simulink model "UserDefinedModel"  (R2023b)
settings: Solver=ode45  StartTime=0.0  StopTime=20  MaxStep=0.001  RelTol=1e-3
libraries: spsSeriesRLCBranchLib x131, spsGroundLib x55, spsCurrentMeasurementLib x48, spsVoltageMeasurementLib x17, spsDiodeLib x4, spsControlledVoltageSourceLib x2, spspowerguiLib x1
(part 1 of 2)
settings Model: Creator=DJJ  LastModifiedBy=HP
settings SolverCC: AlgebraicLoopSolver=TrustRegion
settings DataIOCC: ReturnWorkspaceOutputs=off
settings DebuggingCC: UnconnectedInputMsg=warning  UnconnectedOutputMsg=warning  UnconnectedLineMsg=warning  ArithmeticOperatorsInVariantConditions=warning
settings ModelReferenceCC: EnableRefExpFcnMdlSchedulingChecks=on
settings SFSimCC: CustomCodeUndefinedFunction=UseInterfaceOnly

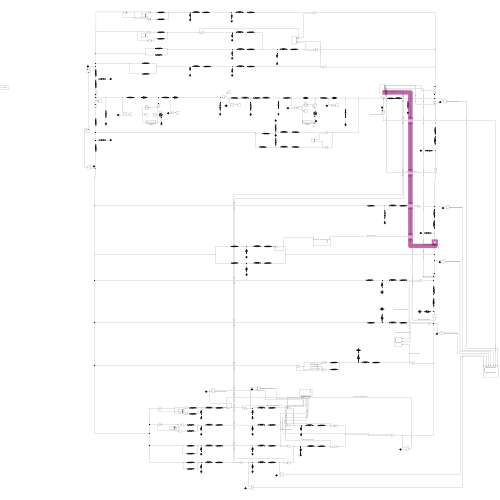
[thumbnail: Simulink's stored preview of the top-level diagram]
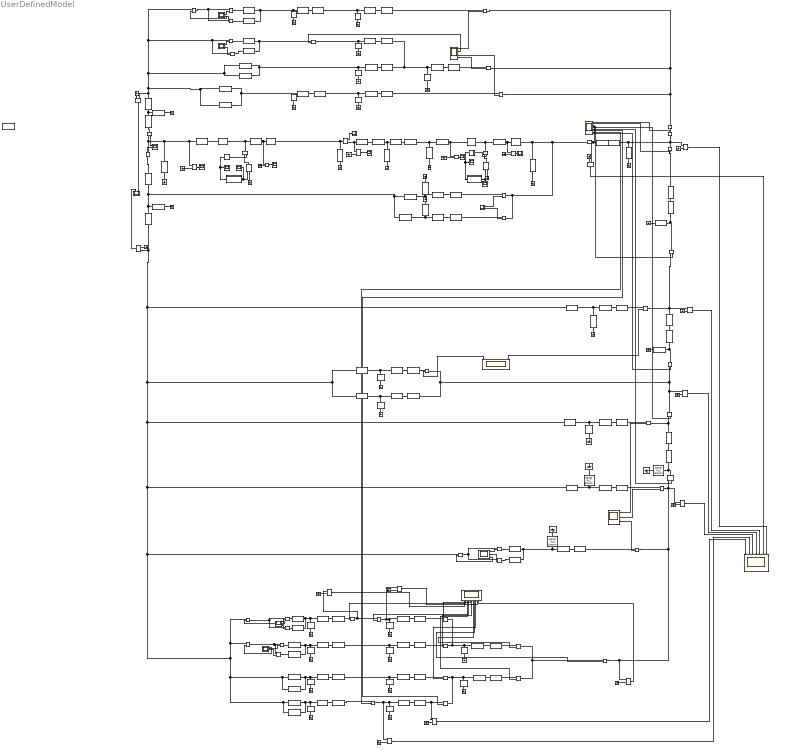
== system UserDefinedModel ==
  Controlled Voltage Source : spsControlledVoltageSourceLib/Controlled Voltage Source  Initialize=off  Source_Type=DC  Amplitude=0  Phase=0  Frequency=0  Measurements=Voltage
  Controlled Voltage Source1 : spsControlledVoltageSourceLib/Controlled Voltage Source  Initialize=off  Source_Type=DC  Amplitude=0  Phase=0  Frequency=0  Measurements=None
  Current Measurement{1,5..19,23..26,31..40,46..49,51..52,58..64,67..68} (45 alike) : spsCurrentMeasurementLib/Current Measurement  PhasorSimulation=off  OutputType=Complex  PSBequivalent=0
  Current Measurement2 : spsCurrentMeasurementLib/Current Measurement  PhasorSimulation=off  OutputType=Magnitude  PSBequivalent=0
  Current Measurement3 : spsCurrentMeasurementLib/Current Measurement  PhasorSimulation=off  OutputType=Magnitude  PSBequivalent=0
  Current Measurement4 : spsCurrentMeasurementLib/Current Measurement  PhasorSimulation=off  OutputType=Magnitude  PSBequivalent=0
  Diode1 : spsDiodeLib/Diode  Ron=0  Lon=0  Vf=0  IC=0  UseSnubber=0  Rs=inf  Cs=250e-9  Measurements=off
  Diode3 : spsDiodeLib/Diode  Ron=0.015  Lon=0  Vf=0  IC=0  UseSnubber=0  Rs=inf  Cs=250e-9  Measurements=off
  Diode5 : spsDiodeLib/Diode  Ron=0  Lon=0  Vf=0  IC=0  UseSnubber=0  Rs=inf  Cs=250e-9  Measurements=off
  Diode7 : spsDiodeLib/Diode  Ron=0.003751  Lon=0  Vf=0  IC=0  UseSnubber=0  Rs=inf  Cs=250e-9  Measurements=off
  Ground{1..30,34,36..40,42..43,47..51,54..55,58..67} (55 alike) : spsGroundLib/Ground  LConnTagsString=a
  Scope1 : Scope  NumInputPorts=5
  Scope{3,5..13} (10 alike) : Scope
  Scope14 : Scope  NumInputPorts=8
  Scope15 : Scope  NumInputPorts=2
  Scope16 : Scope  NumInputPorts=3
  Scope18 : Scope  NumInputPorts=11
  Scope2 : Scope  NumInputPorts=9
  Scope20 : Scope  NumInputPorts=3
  Scope21 : Scope  NumInputPorts=2
  Scope22 : Scope  NumInputPorts=5
  Scope23 : Scope  NumInputPorts=6
  Scope26 : Scope  NumInputPorts=7
  Scope27 : Scope  NumInputPorts=7
  Scope28 : Scope  NumInputPorts=3
  Scope4 : Scope  NumInputPorts=7
  Series RLC Branch1 : spsSeriesRLCBranchLib/Series RLC Branch  LConnTagsString=__new0  RConnTagsString=__new0  BranchType=R  Resistance=0.05  Inductance=1e-3  SetiL0=off  InitialCurrent=0  Capacitance=1e-6  Setx0=off  InitialVoltage=0  Measurements=None
  Series RLC Branch10 : spsSeriesRLCBranchLib/Series RLC Branch  LConnTagsString=__new0  RConnTagsString=__new0  BranchType=R  Resistance=0.025  Inductance=1e-3  SetiL0=off  InitialCurrent=0  Capacitance=1e-6  Setx0=off  InitialVoltage=0  Measurements=None
  Series RLC Branch11 : spsSeriesRLCBranchLib/Series RLC Branch  LConnTagsString=__new0  RConnTagsString=__new0  BranchType=L  Resistance=1  Inductance=0.001  SetiL0=off  InitialCurrent=0  Capacitance=1e-6  Setx0=off  InitialVoltage=0  Measurements=None
  Series RLC Branch110 : spsSeriesRLCBranchLib/Series RLC Branch  LConnTagsString=__new0  RConnTagsString=__new0  BranchType=R  Resistance=16.45  Inductance=1e-3  SetiL0=off  InitialCurrent=0  Capacitance=1e-6  Setx0=off  InitialVoltage=0  Measurements=None
  Series RLC Branch111 : spsSeriesRLCBranchLib/Series RLC Branch  LConnTagsString=__new0  RConnTagsString=__new0  BranchType=R  Resistance=2.5  Inductance=1e-3  SetiL0=off  InitialCurrent=0  Capacitance=1e-6  Setx0=off  InitialVoltage=0  Measurements=None
  Series RLC Branch{51,112,116,121} (4 alike) : spsSeriesRLCBranchLib/Series RLC Branch  LConnTagsString=__new0  RConnTagsString=__new0  BranchType=L  Resistance=1  Inductance=0.12  SetiL0=off  InitialCurrent=0  Capacitance=1e-6  Setx0=off  InitialVoltage=0  Measurements=None
  Series RLC Branch113 : spsSeriesRLCBranchLib/Series RLC Branch  LConnTagsString=__new0  RConnTagsString=__new0  BranchType=C  Resistance=1  Inductance=1e-3  SetiL0=off  InitialCurrent=0  Capacitance=0.05  Setx0=off  InitialVoltage=0  Measurements=None
  Series RLC Branch114 : spsSeriesRLCBranchLib/Series RLC Branch  LConnTagsString=__new0  RConnTagsString=__new0  BranchType=R  Resistance=16.45  Inductance=1e-3  SetiL0=off  InitialCurrent=0  Capacitance=1e-6  Setx0=off  InitialVoltage=0  Measurements=None
  Series RLC Branch115 : spsSeriesRLCBranchLib/Series RLC Branch  LConnTagsString=__new0  RConnTagsString=__new0  BranchType=R  Resistance=2.5  Inductance=1e-3  SetiL0=off  InitialCurrent=0  Capacitance=1e-6  Setx0=off  InitialVoltage=0  Measurements=None
  Series RLC Branch117 : spsSeriesRLCBranchLib/Series RLC Branch  LConnTagsString=__new0  RConnTagsString=__new0  BranchType=C  Resistance=1  Inductance=1e-3  SetiL0=off  InitialCurrent=0  Capacitance=0.05  Setx0=off  InitialVoltage=0  Measurements=None
  Series RLC Branch118 : spsSeriesRLCBranchLib/Series RLC Branch  LConnTagsString=__new0  RConnTagsString=__new0  BranchType=R  Resistance=0.07  Inductance=1e-3  SetiL0=off  InitialCurrent=0  Capacitance=1e-6  Setx0=off  InitialVoltage=0  Measurements=None
  Series RLC Branch119 : spsSeriesRLCBranchLib/Series RLC Branch  LConnTagsString=__new0  RConnTagsString=__new0  BranchType=L  Resistance=1  Inductance=0.0028  SetiL0=off  InitialCurrent=0  Capacitance=1e-6  Setx0=off  InitialVoltage=0  Measurements=None
  Series RLC Branch12 : spsSeriesRLCBranchLib/Series RLC Branch  LConnTagsString=__new0  RConnTagsString=__new0  BranchType=C  Resistance=1  Inductance=1e-3  SetiL0=off  InitialCurrent=0  Capacitance=3  Setx0=on  InitialVoltage=13.392  Measurements=None
  Series RLC Branch120 : spsSeriesRLCBranchLib/Series RLC Branch  LConnTagsString=__new0  RConnTagsString=__new0  BranchType=R  Resistance=1.5  Inductance=1e-3  SetiL0=off  InitialCurrent=0  Capacitance=1e-6  Setx0=off  InitialVoltage=0  Measurements=None
  Series RLC Branch122 : spsSeriesRLCBranchLib/Series RLC Branch  LConnTagsString=__new0  RConnTagsString=__new0  BranchType=C  Resistance=1  Inductance=1e-3  SetiL0=off  InitialCurrent=0  Capacitance=0.05  Setx0=off  InitialVoltage=0  Measurements=None
  Series RLC Branch123 : spsSeriesRLCBranchLib/Series RLC Branch  LConnTagsString=__new0  RConnTagsString=__new0  BranchType=R  Resistance=7.05  Inductance=1e-3  SetiL0=off  InitialCurrent=0  Capacitance=1e-6  Setx0=off  InitialVoltage=0  Measurements=None
  Series RLC Branch124 : spsSeriesRLCBranchLib/Series RLC Branch  LConnTagsString=__new0  RConnTagsString=__new0  BranchType=C  Resistance=1  Inductance=1e-3  SetiL0=off  InitialCurrent=0  Capacitance=0.1  Setx0=off  InitialVoltage=0  Measurements=None
  Series RLC Branch125 : spsSeriesRLCBranchLib/Series RLC Branch  LConnTagsString=__new0  RConnTagsString=__new0  BranchType=R  Resistance=4  Inductance=1e-3  SetiL0=off  InitialCurrent=0  Capacitance=1e-6  Setx0=off  InitialVoltage=0  Measurements=None
  Series RLC Branch126 : spsSeriesRLCBranchLib/Series RLC Branch  LConnTagsString=__new0  RConnTagsString=__new0  BranchType=L  Resistance=1  Inductance=0.36  SetiL0=off  InitialCurrent=0  Capacitance=1e-6  Setx0=off  InitialVoltage=0  Measurements=None
  Series RLC Branch127 : spsSeriesRLCBranchLib/Series RLC Branch  LConnTagsString=__new0  RConnTagsString=__new0  BranchType=C  Resistance=1  Inductance=1e-3  SetiL0=off  InitialCurrent=0  Capacitance=0.01  Setx0=off  InitialVoltage=0  Measurements=None
  Series RLC Branch128 : spsSeriesRLCBranchLib/Series RLC Branch  LConnTagsString=__new0  RConnTagsString=__new0  BranchType=R  Resistance=47  Inductance=1e-3  SetiL0=off  InitialCurrent=0  Capacitance=1e-6  Setx0=off  InitialVoltage=0  Measurements=None
  Series RLC Branch129 : spsSeriesRLCBranchLib/Series RLC Branch  LConnTagsString=__new0  RConnTagsString=__new0  BranchType=R  Resistance=54.58204  Inductance=1e-3  SetiL0=off  InitialCurrent=0  Capacitance=1e-6  Setx0=off  InitialVoltage=0  Measurements=None
  Series RLC Branch{5,19,87,132} (4 alike) : spsSeriesRLCBranchLib/Series RLC Branch  LConnTagsString=__new0  RConnTagsString=__new0  BranchType=R  Resistance=0.3  Inductance=1e-3  SetiL0=off  InitialCurrent=0  Capacitance=1e-6  Setx0=off  InitialVoltage=0  Measurements=None
  Series RLC Branch133 : spsSeriesRLCBranchLib/Series RLC Branch  LConnTagsString=__new0  RConnTagsString=__new0  BranchType=L  Resistance=1  Inductance=0.04  SetiL0=off  InitialCurrent=0  Capacitance=1e-6  Setx0=off  InitialVoltage=0  Measurements=None
  Series RLC Branch135 : spsSeriesRLCBranchLib/Series RLC Branch  LConnTagsString=__new0  RConnTagsString=__new0  BranchType=R  Resistance=143.364  Inductance=1e-3  SetiL0=off  InitialCurrent=0  Capacitance=1e-6  Setx0=off  InitialVoltage=0  Measurements=None
  Series RLC Branch136 : spsSeriesRLCBranchLib/Series RLC Branch  LConnTagsString=__new0  RConnTagsString=__new0  BranchType=R  Resistance=1.5  Inductance=1e-3  SetiL0=off  InitialCurrent=0  Capacitance=1e-6  Setx0=off  InitialVoltage=0  Measurements=None
  Series RLC Branch137 : spsSeriesRLCBranchLib/Series RLC Branch  LConnTagsString=__new0  RConnTagsString=__new0  BranchType=L  Resistance=1  Inductance=0.028  SetiL0=off  InitialCurrent=0  Capacitance=1e-6  Setx0=off  InitialVoltage=0  Measurements=None
  Series RLC Branch{7,138..139,143} (4 alike) : spsSeriesRLCBranchLib/Series RLC Branch  LConnTagsString=__new0  RConnTagsString=__new0  BranchType=C  Resistance=1  Inductance=1e-3  SetiL0=off  InitialCurrent=0  Capacitance=0.009  Setx0=off  InitialVoltage=0  Measurements=None
  Series RLC Branch14 : spsSeriesRLCBranchLib/Series RLC Branch  LConnTagsString=__new0  RConnTagsString=__new0  BranchType=R  Resistance=21.889  Inductance=1e-3  SetiL0=off  InitialCurrent=0  Capacitance=1e-6  Setx0=off  InitialVoltage=0  Measurements=None
  Series RLC Branch140 : spsSeriesRLCBranchLib/Series RLC Branch  LConnTagsString=__new0  RConnTagsString=__new0  BranchType=R  Resistance=143.364  Inductance=1e-3  SetiL0=off  InitialCurrent=0  Capacitance=1e-6  Setx0=off  InitialVoltage=0  Measurements=None
  Series RLC Branch141 : spsSeriesRLCBranchLib/Series RLC Branch  LConnTagsString=__new0  RConnTagsString=__new0  BranchType=R  Resistance=1.5  Inductance=1e-3  SetiL0=off  InitialCurrent=0  Capacitance=1e-6  Setx0=off  InitialVoltage=0  Measurements=None
  Series RLC Branch142 : spsSeriesRLCBranchLib/Series RLC Branch  LConnTagsString=__new0  RConnTagsString=__new0  BranchType=L  Resistance=1  Inductance=0.028  SetiL0=off  InitialCurrent=0  Capacitance=1e-6  Setx0=off  InitialVoltage=0  Measurements=None
  Series RLC Branch15 : spsSeriesRLCBranchLib/Series RLC Branch  LConnTagsString=__new0  RConnTagsString=__new0  BranchType=C  Resistance=1  Inductance=1e-3  SetiL0=off  InitialCurrent=0  Capacitance=0.038  Setx0=off  InitialVoltage=0  Measurements=None
  Series RLC Branch150 : spsSeriesRLCBranchLib/Series RLC Branch  LConnTagsString=__new0  RConnTagsString=__new0  BranchType=R  Resistance=21.889  Inductance=1e-3  SetiL0=off  InitialCurrent=0  Capacitance=1e-6  Setx0=off  InitialVoltage=0  Measurements=None
  Series RLC Branch151 : spsSeriesRLCBranchLib/Series RLC Branch  LConnTagsString=__new0  RConnTagsString=__new0  BranchType=R  Resistance=48.3677  Inductance=1e-3  SetiL0=off  InitialCurrent=0  Capacitance=1e-6  Setx0=off  InitialVoltage=0  Measurements=None
  Series RLC Branch{152,158,160,164,167,177} (6 alike) : spsSeriesRLCBranchLib/Series RLC Branch  LConnTagsString=__new0  RConnTagsString=__new0  BranchType=R  Resistance=2  Inductance=1e-3  SetiL0=off  InitialCurrent=0  Capacitance=1e-6  Setx0=off  InitialVoltage=0  Measurements=None
  Series RLC Branch153 : spsSeriesRLCBranchLib/Series RLC Branch  LConnTagsString=__new0  RConnTagsString=__new0  BranchType=L  Resistance=1  Inductance=0.03  SetiL0=off  InitialCurrent=0  Capacitance=1e-6  Setx0=off  InitialVoltage=0  Measurements=None
  Series RLC Branch154 : spsSeriesRLCBranchLib/Series RLC Branch  LConnTagsString=__new0  RConnTagsString=__new0  BranchType=C  Resistance=1  Inductance=1e-3  SetiL0=off  InitialCurrent=0  Capacitance=0.018  Setx0=off  InitialVoltage=0  Measurements=None
  Series RLC Branch155 : spsSeriesRLCBranchLib/Series RLC Branch  LConnTagsString=__new0  RConnTagsString=__new0  BranchType=R  Resistance=126.5632  Inductance=1e-3  SetiL0=off  InitialCurrent=0  Capacitance=1e-6  Setx0=off  InitialVoltage=0  Measurements=None
  Series RLC Branch159 : spsSeriesRLCBranchLib/Series RLC Branch  LConnTagsString=__new0  RConnTagsString=__new0  BranchType=L  Resistance=1  Inductance=0.15  SetiL0=off  InitialCurrent=0  Capacitance=1e-6  Setx0=off  InitialVoltage=0  Measurements=None
  Series RLC Branch16 : spsSeriesRLCBranchLib/Series RLC Branch  LConnTagsString=__new0  RConnTagsString=__new0  BranchType=R  Resistance=0.35  Inductance=1e-3  SetiL0=off  InitialCurrent=0  Capacitance=1e-6  Setx0=off  InitialVoltage=0  Measurements=None
  Series RLC Branch161 : spsSeriesRLCBranchLib/Series RLC Branch  LConnTagsString=__new0  RConnTagsString=__new0  BranchType=L  Resistance=1  Inductance=0.25  SetiL0=off  InitialCurrent=0  Capacitance=1e-6  Setx0=off  InitialVoltage=0  Measurements=None
  Series RLC Branch162 : spsSeriesRLCBranchLib/Series RLC Branch  LConnTagsString=__new0  RConnTagsString=__new0  BranchType=C  Resistance=1  Inductance=1e-3  SetiL0=off  InitialCurrent=0  Capacitance=0.006  Setx0=off  InitialVoltage=0  Measurements=None
  Series RLC Branch{74,78,94,163,166} (5 alike) : spsSeriesRLCBranchLib/Series RLC Branch  LConnTagsString=__new0  RConnTagsString=__new0  BranchType=C  Resistance=1  Inductance=1e-3  SetiL0=off  InitialCurrent=0  Capacitance=0.005  Setx0=off  InitialVoltage=0  Measurements=None
  Series RLC Branch165 : spsSeriesRLCBranchLib/Series RLC Branch  LConnTagsString=__new0  RConnTagsString=__new0  BranchType=L  Resistance=1  Inductance=0.25  SetiL0=off  InitialCurrent=0  Capacitance=1e-6  Setx0=off  InitialVoltage=0  Measurements=None
  Series RLC Branch168 : spsSeriesRLCBranchLib/Series RLC Branch  LConnTagsString=__new0  RConnTagsString=__new0  BranchType=L  Resistance=1  Inductance=0.15  SetiL0=off  InitialCurrent=0  Capacitance=1e-6  Setx0=off  InitialVoltage=0  Measurements=None
  Series RLC Branch169 : spsSeriesRLCBranchLib/Series RLC Branch  LConnTagsString=__new0  RConnTagsString=__new0  BranchType=C  Resistance=1  Inductance=1e-3  SetiL0=off  InitialCurrent=0  Capacitance=0.006  Setx0=off  InitialVoltage=0  Measurements=None
  Series RLC Branch17 : spsSeriesRLCBranchLib/Series RLC Branch  LConnTagsString=__new0  RConnTagsString=__new0  BranchType=L  Resistance=1  Inductance=0.06  SetiL0=off  InitialCurrent=0  Capacitance=1e-6  Setx0=off  InitialVoltage=0  Measurements=None
  Series RLC Branch170 : spsSeriesRLCBranchLib/Series RLC Branch  LConnTagsString=__new0  RConnTagsString=__new0  BranchType=R  Resistance=0.05  Inductance=1e-3  SetiL0=off  InitialCurrent=0  Capacitance=1e-6  Setx0=off  InitialVoltage=0  Measurements=None
  Series RLC Branch171 : spsSeriesRLCBranchLib/Series RLC Branch  LConnTagsString=__new0  RConnTagsString=__new0  BranchType=L  Resistance=1  Inductance=0.004  SetiL0=off  InitialCurrent=0  Capacitance=1e-6  Setx0=off  InitialVoltage=0  Measurements=None
  Series RLC Branch172 : spsSeriesRLCBranchLib/Series RLC Branch  LConnTagsString=__new0  RConnTagsString=__new0  BranchType=C  Resistance=1  Inductance=1e-3  SetiL0=off  InitialCurrent=0  Capacitance=0.012  Setx0=off  InitialVoltage=0  Measurements=None
  Series RLC Branch173 : spsSeriesRLCBranchLib/Series RLC Branch  LConnTagsString=__new0  RConnTagsString=__new0  BranchType=R  Resistance=0.05  Inductance=1e-3  SetiL0=off  InitialCurrent=0  Capacitance=1e-6  Setx0=off  InitialVoltage=0  Measurements=None
  Series RLC Branch174 : spsSeriesRLCBranchLib/Series RLC Branch  LConnTagsString=__new0  RConnTagsString=__new0  BranchType=L  Resistance=1  Inductance=0.004  SetiL0=off  InitialCurrent=0  Capacitance=1e-6  Setx0=off  InitialVoltage=0  Measurements=None
  Series RLC Branch175 : spsSeriesRLCBranchLib/Series RLC Branch  LConnTagsString=__new0  RConnTagsString=__new0  BranchType=C  Resistance=1  Inductance=1e-3  SetiL0=off  InitialCurrent=0  Capacitance=0.012  Setx0=off  InitialVoltage=0  Measurements=None
  Series RLC Branch176 : spsSeriesRLCBranchLib/Series RLC Branch  LConnTagsString=__new0  RConnTagsString=__new0  BranchType=R  Resistance=67.5  Inductance=1e-3  SetiL0=off  InitialCurrent=0  Capacitance=1e-6  Setx0=off  InitialVoltage=0  Measurements=None
  Series RLC Branch178 : spsSeriesRLCBranchLib/Series RLC Branch  LConnTagsString=__new0  RConnTagsString=__new0  BranchType=C  Resistance=1  Inductance=1e-3  SetiL0=off  InitialCurrent=0  Capacitance=0.0012  Setx0=off  InitialVoltage=0  Measurements=None
  Series RLC Branch179 : spsSeriesRLCBranchLib/Series RLC Branch  LConnTagsString=__new0  RConnTagsString=__new0  BranchType=L  Resistance=1  Inductance=3.5  SetiL0=off  InitialCurrent=0  Capacitance=1e-6  Setx0=off  InitialVoltage=0  Measurements=None
  Series RLC Branch18 : spsSeriesRLCBranchLib/Series RLC Branch  LConnTagsString=__new0  RConnTagsString=__new0  BranchType=R  Resistance=35.84  Inductance=1e-3  SetiL0=off  InitialCurrent=0  Capacitance=1e-6  Setx0=off  InitialVoltage=0  Measurements=None
  Series RLC Branch180 : spsSeriesRLCBranchLib/Series RLC Branch  LConnTagsString=__new0  RConnTagsString=__new0  BranchType=R  Resistance=21.15  Inductance=1e-3  SetiL0=off  InitialCurrent=0  Capacitance=1e-6  Setx0=off  InitialVoltage=0  Measurements=None
  Series RLC Branch186 : spsSeriesRLCBranchLib/Series RLC Branch  LConnTagsString=__new0  RConnTagsString=__new0  BranchType=R  Resistance=61.55214  Inductance=1e-3  SetiL0=off  InitialCurrent=0  Capacitance=1e-6  Setx0=off  InitialVoltage=0  Measurements=None
  Series RLC Branch187 : spsSeriesRLCBranchLib/Series RLC Branch  LConnTagsString=__new0  RConnTagsString=__new0  BranchType=R  Resistance=17.6218  Inductance=1e-3  SetiL0=off  InitialCurrent=0  Capacitance=1e-6  Setx0=off  InitialVoltage=0  Measurements=None
  Series RLC Branch2 : spsSeriesRLCBranchLib/Series RLC Branch  LConnTagsString=__new0  RConnTagsString=__new0  BranchType=L  Resistance=1  Inductance=0.0015  SetiL0=on  InitialCurrent=23.836  Capacitance=1e-6  Setx0=off  InitialVoltage=0  Measurements=None
  Series RLC Branch20 : spsSeriesRLCBranchLib/Series RLC Branch  LConnTagsString=__new0  RConnTagsString=__new0  BranchType=L  Resistance=1  Inductance=0.005  SetiL0=off  InitialCurrent=0  Capacitance=1e-6  Setx0=off  InitialVoltage=0  Measurements=None
  Series RLC Branch21 : spsSeriesRLCBranchLib/Series RLC Branch  LConnTagsString=__new0  RConnTagsString=__new0  BranchType=C  Resistance=1  Inductance=1e-3  SetiL0=off  InitialCurrent=0  Capacitance=0.012  Setx0=off  InitialVoltage=0  Measurements=None
  Series RLC Branch22 : spsSeriesRLCBranchLib/Series RLC Branch  LConnTagsString=__new0  RConnTagsString=__new0  BranchType=R  Resistance=0.015  Inductance=1e-3  SetiL0=off  InitialCurrent=0  Capacitance=1e-6  Setx0=off  InitialVoltage=0  Measurements=None
  Series RLC Branch24 : spsSeriesRLCBranchLib/Series RLC Branch  LConnTagsString=__new0  RConnTagsString=__new0  BranchType=R  Resistance=0.03  Inductance=1e-3  SetiL0=off  InitialCurrent=0  Capacitance=1e-6  Setx0=off  InitialVoltage=0  Measurements=None
  Series RLC Branch25 : spsSeriesRLCBranchLib/Series RLC Branch  LConnTagsString=__new0  RConnTagsString=__new0  BranchType=R  Resistance=0.003751  Inductance=1e-3  SetiL0=off  InitialCurrent=0  Capacitance=1e-6  Setx0=off  InitialVoltage=0  Measurements=None
  Series RLC Branch26 : spsSeriesRLCBranchLib/Series RLC Branch  LConnTagsString=__new0  RConnTagsString=__new0  BranchType=L  Resistance=1  Inductance=0.0012  SetiL0=off  InitialCurrent=0  Capacitance=1e-6  Setx0=off  InitialVoltage=0  Measurements=None
  Series RLC Branch27 : spsSeriesRLCBranchLib/Series RLC Branch  LConnTagsString=__new0  RConnTagsString=__new0  BranchType=C  Resistance=1  Inductance=1e-3  SetiL0=off  InitialCurrent=0  Capacitance=0.2  Setx0=off  InitialVoltage=0  Measurements=None
  Series RLC Branch28 : spsSeriesRLCBranchLib/Series RLC Branch  LConnTagsString=__new0  RConnTagsString=__new0  BranchType=C  Resistance=1  Inductance=1e-3  SetiL0=off  InitialCurrent=0  Capacitance=46.7  Setx0=on  InitialVoltage=11.295  Measurements=Branch voltage
  Series RLC Branch3 : spsSeriesRLCBranchLib/Series RLC Branch  LConnTagsString=__new0  RConnTagsString=__new0  BranchType=R  Resistance=36  Inductance=1e-3  SetiL0=off  InitialCurrent=0  Capacitance=1e-6  Setx0=off  InitialVoltage=0  Measurements=None
  Series RLC Branch31 : spsSeriesRLCBranchLib/Series RLC Branch  LConnTagsString=__new0  RConnTagsString=__new0  BranchType=C  Resistance=1  Inductance=1e-3  SetiL0=off  InitialCurrent=0  Capacitance=0.03  Setx0=on  InitialVoltage=0  Measurements=None
  Series RLC Branch{32,43,69..70,84,91} (6 alike) : spsSeriesRLCBranchLib/Series RLC Branch  LConnTagsString=__new0  RConnTagsString=__new0  BranchType=R  Resistance=0.001  Inductance=1e-3  SetiL0=off  InitialCurrent=0  Capacitance=1e-6  Setx0=off  InitialVoltage=0  Measurements=None
  Series RLC Branch33 : spsSeriesRLCBranchLib/Series RLC Branch  LConnTagsString=__new0  RConnTagsString=__new0  BranchType=L  Resistance=1  Inductance=0.00003  SetiL0=off  InitialCurrent=0  Capacitance=1e-6  Setx0=off  InitialVoltage=0  Measurements=None
  Series RLC Branch34 : spsSeriesRLCBranchLib/Series RLC Branch  LConnTagsString=__new0  RConnTagsString=__new0  BranchType=C  Resistance=1  Inductance=1e-3  SetiL0=off  InitialCurrent=0  Capacitance=0.4  Setx0=off  InitialVoltage=0  Measurements=None
  Series RLC Branch4 : spsSeriesRLCBranchLib/Series RLC Branch  LConnTagsString=__new0  RConnTagsString=__new0  BranchType=R  Resistance=54.58204  Inductance=1e-3  SetiL0=off  InitialCurrent=0  Capacitance=1e-6  Setx0=off  InitialVoltage=0  Measurements=None
  Series RLC Branch42 : spsSeriesRLCBranchLib/Series RLC Branch  LConnTagsString=__new0  RConnTagsString=__new0  BranchType=R  Resistance=0.03  Inductance=1e-3  SetiL0=off  InitialCurrent=0  Capacitance=1e-6  Setx0=off  InitialVoltage=0  Measurements=None
  Series RLC Branch44 : spsSeriesRLCBranchLib/Series RLC Branch  LConnTagsString=__new0  RConnTagsString=__new0  BranchType=R  Resistance=0.025  Inductance=1e-3  SetiL0=off  InitialCurrent=0  Capacitance=1e-6  Setx0=off  InitialVoltage=0  Measurements=None
  Series RLC Branch45 : spsSeriesRLCBranchLib/Series RLC Branch  LConnTagsString=__new0  RConnTagsString=__new0  BranchType=R  Resistance=0.01  Inductance=1e-3  SetiL0=off  InitialCurrent=0  Capacitance=1e-6  Setx0=off  InitialVoltage=0  Measurements=None
  Series RLC Branch46 : spsSeriesRLCBranchLib/Series RLC Branch  LConnTagsString=__new0  RConnTagsString=__new0  BranchType=L  Resistance=1  Inductance=0.0018  SetiL0=off  InitialCurrent=0  Capacitance=1e-6  Setx0=off  InitialVoltage=0  Measurements=None
  Series RLC Branch47 : spsSeriesRLCBranchLib/Series RLC Branch  LConnTagsString=__new0  RConnTagsString=__new0  BranchType=C  Resistance=1  Inductance=1e-3  SetiL0=off  InitialCurrent=0  Capacitance=0.15  Setx0=off  InitialVoltage=0  Measurements=None
  Series RLC Branch48 : spsSeriesRLCBranchLib/Series RLC Branch  LConnTagsString=__new0  RConnTagsString=__new0  BranchType=C  Resistance=1  Inductance=1e-3  SetiL0=off  InitialCurrent=0  Capacitance=0.25  Setx0=off  InitialVoltage=0  Measurements=None
  Series RLC Branch49 : spsSeriesRLCBranchLib/Series RLC Branch  LConnTagsString=__new0  RConnTagsString=__new0  BranchType=C  Resistance=1  Inductance=1e-3  SetiL0=off  InitialCurrent=0  Capacitance=0.06  Setx0=off  InitialVoltage=0  Measurements=None
  Series RLC Branch50 : spsSeriesRLCBranchLib/Series RLC Branch  LConnTagsString=__new0  RConnTagsString=__new0  BranchType=R  Resistance=1  Inductance=1e-3  SetiL0=off  InitialCurrent=0  Capacitance=1e-6  Setx0=off  InitialVoltage=0  Measurements=None
  Series RLC Branch54 : spsSeriesRLCBranchLib/Series RLC Branch  LConnTagsString=__new0  RConnTagsString=__new0  BranchType=R  Resistance=21.15  Inductance=1e-3  SetiL0=off  InitialCurrent=0  Capacitance=1e-6  Setx0=off  InitialVoltage=0  Measurements=None
  Series RLC Branch55 : spsSeriesRLCBranchLib/Series RLC Branch  LConnTagsString=__new0  RConnTagsString=__new0  BranchType=R  Resistance=48.3677  Inductance=1e-3  SetiL0=off  InitialCurrent=0  Capacitance=1e-6  Setx0=off  InitialVoltage=0  Measurements=None
  Series RLC Branch58 : spsSeriesRLCBranchLib/Series RLC Branch  LConnTagsString=__new0  RConnTagsString=__new0  BranchType=R  Resistance=39.715  Inductance=1e-3  SetiL0=off  InitialCurrent=0  Capacitance=1e-6  Setx0=off  InitialVoltage=0  Measurements=None
  Series RLC Branch59 : spsSeriesRLCBranchLib/Series RLC Branch  LConnTagsString=__new0  RConnTagsString=__new0  BranchType=R  Resistance=17.6218  Inductance=1e-3  SetiL0=off  InitialCurrent=0  Capacitance=1e-6  Setx0=off  InitialVoltage=0  Measurements=None
  Series RLC Branch6 : spsSeriesRLCBranchLib/Series RLC Branch  LConnTagsString=__new0  RConnTagsString=__new0  BranchType=L  Resistance=1  Inductance=0.04  SetiL0=off  InitialCurrent=0  Capacitance=1e-6  Setx0=off  InitialVoltage=0  Measurements=None
  Series RLC Branch60 : spsSeriesRLCBranchLib/Series RLC Branch  LConnTagsString=__new0  RConnTagsString=__new0  BranchType=R  Resistance=61.55214  Inductance=1e-3  SetiL0=off  InitialCurrent=0  Capacitance=1e-6  Setx0=off  InitialVoltage=0  Measurements=None
  Series RLC Branch61 : spsSeriesRLCBranchLib/Series RLC Branch  LConnTagsString=__new0  RConnTagsString=__new0  BranchType=R  Resistance=7.05  Inductance=1e-3  SetiL0=off  InitialCurrent=0  Capacitance=1e-6  Setx0=off  InitialVoltage=0  Measurements=None
  Series RLC Branch64 : spsSeriesRLCBranchLib/Series RLC Branch  LConnTagsString=__new0  RConnTagsString=__new0  BranchType=R  Resistance=0.0005  Inductance=1e-3  SetiL0=off  InitialCurrent=0  Capacitance=1e-6  Setx0=off  InitialVoltage=0  Measurements=None
  Series RLC Branch65 : spsSeriesRLCBranchLib/Series RLC Branch  LConnTagsString=__new0  RConnTagsString=__new0  BranchType=C  Resistance=1  Inductance=1e-3  SetiL0=off  InitialCurrent=0  Capacitance=7.5  Setx0=off  InitialVoltage=0  Measurements=None
  Series RLC Branch66 : spsSeriesRLCBranchLib/Series RLC Branch  LConnTagsString=__new0  RConnTagsString=__new0  BranchType=R  Resistance=5  Inductance=1e-3  SetiL0=off  InitialCurrent=0  Capacitance=1e-6  Setx0=off  InitialVoltage=0  Measurements=None
  Series RLC Branch67 : spsSeriesRLCBranchLib/Series RLC Branch  LConnTagsString=__new0  RConnTagsString=__new0  BranchType=C  Resistance=1  Inductance=1e-3  SetiL0=off  InitialCurrent=0  Capacitance=0.0035  Setx0=off  InitialVoltage=0  Measurements=None
  Series RLC Branch68 : spsSeriesRLCBranchLib/Series RLC Branch  LConnTagsString=__new0  RConnTagsString=__new0  BranchType=L  Resistance=1  Inductance=0.0005  SetiL0=off  InitialCurrent=0  Capacitance=1e-6  Setx0=off  InitialVoltage=0  Measurements=None
  Series RLC Branch71 : spsSeriesRLCBranchLib/Series RLC Branch  LConnTagsString=__new0  RConnTagsString=__new0  BranchType=C  Resistance=1  Inductance=1e-3  SetiL0=off  InitialCurrent=0  Capacitance=5  Setx0=off  InitialVoltage=0  Measurements=None
  Series RLC Branch72 : spsSeriesRLCBranchLib/Series RLC Branch  LConnTagsString=__new0  RConnTagsString=__new0  BranchType=R  Resistance=0.0005  Inductance=1e-3  SetiL0=off  InitialCurrent=0  Capacitance=1e-6  Setx0=off  InitialVoltage=0  Measurements=None
  Series RLC Branch73 : spsSeriesRLCBranchLib/Series RLC Branch  LConnTagsString=__new0  RConnTagsString=__new0  BranchType=R  Resistance=35.84  Inductance=1e-3  SetiL0=off  InitialCurrent=0  Capacitance=1e-6  Setx0=off  InitialVoltage=0  Measurements=None
  Series RLC Branch79 : spsSeriesRLCBranchLib/Series RLC Branch  LConnTagsString=__new0  RConnTagsString=__new0  BranchType=C  Resistance=1  Inductance=1e-3  SetiL0=off  InitialCurrent=0  Capacitance=0.038  Setx0=off  InitialVoltage=0  Measurements=None
  Series RLC Branch8 : spsSeriesRLCBranchLib/Series RLC Branch  LConnTagsString=__new0  RConnTagsString=__new0  BranchType=L  Resistance=1  Inductance=2  SetiL0=off  InitialCurrent=0  Capacitance=1e-6  Setx0=off  InitialVoltage=0  Measurements=None
  Series RLC Branch80 : spsSeriesRLCBranchLib/Series RLC Branch  LConnTagsString=__new0  RConnTagsString=__new0  BranchType=R  Resistance=0.35  Inductance=1e-3  SetiL0=off  InitialCurrent=0  Capacitance=1e-6  Setx0=off  InitialVoltage=0  Measurements=None
  Series RLC Branch81 : spsSeriesRLCBranchLib/Series RLC Branch  LConnTagsString=__new0  RConnTagsString=__new0  BranchType=L  Resistance=1  Inductance=0.06  SetiL0=off  InitialCurrent=0  Capacitance=1e-6  Setx0=off  InitialVoltage=0  Measurements=None
  Series RLC Branch85 : spsSeriesRLCBranchLib/Series RLC Branch  LConnTagsString=__new0  RConnTagsString=__new0  BranchType=L  Resistance=1  Inductance=0.0005  SetiL0=off  InitialCurrent=0  Capacitance=1e-6  Setx0=off  InitialVoltage=0  Measurements=None
  Series RLC Branch88 : spsSeriesRLCBranchLib/Series RLC Branch  LConnTagsString=__new0  RConnTagsString=__new0  BranchType=L  Resistance=1  Inductance=0.005  SetiL0=off  InitialCurrent=0  Capacitance=1e-6  Setx0=off  InitialVoltage=0  Measurements=None
  Series RLC Branch9 : spsSeriesRLCBranchLib/Series RLC Branch  LConnTagsString=__new0  RConnTagsString=__new0  BranchType=C  Resistance=1  Inductance=1e-3  SetiL0=off  InitialCurrent=0  Capacitance=20  Setx0=on  InitialVoltage=3.3268  Measurements=None
  Series RLC Branch92 : spsSeriesRLCBranchLib/Series RLC Branch  LConnTagsString=__new0  RConnTagsString=__new0  BranchType=C  Resistance=1  Inductance=1e-3  SetiL0=off  InitialCurrent=0  Capacitance=0.02  Setx0=off  InitialVoltage=0  Measurements=None
  Series RLC Branch93 : spsSeriesRLCBranchLib/Series RLC Branch  LConnTagsString=__new0  RConnTagsString=__new0  BranchType=L  Resistance=1  Inductance=0.0005  SetiL0=off  InitialCurrent=0  Capacitance=1e-6  Setx0=off  InitialVoltage=0  Measurements=None
  Voltage Measurement{1..17} (17 alike) : spsVoltageMeasurementLib/Voltage Measurement  PhasorSimulation=off  OutputType=Complex  PSBequivalent=0
  capbianlv : Subsystem
  capbianlv1 : Subsystem
  inter : Subsystem
  inter1 : Subsystem
  powergui : spspowerguiLib/powergui  Priority=1  SimulationMode=Continuous  SampleTime=0.00001  frequency=60  Iterations=50  frequencyindice=0  Pbase=100e6  ErrMax=1e-4  UnitsV=kV  UnitsW=MW  buscounter=0  FunctionMessages=off  echomessages=off  EnableUseOfTLC=off  CurrentSourceSwitches=off  DisableSnubberDevices=off  DisableRonSwitches=off  DisableVfSwitches=off  DisplayEquations=off  AutomaticDiscreteSolvers=off  SolverType=Tustin/Backward Euler (TBE)  Interpol=off  ExternalGateDelay=off  methode=off  Ts=100  x0status=blocks  SPID=off  SwTol=0  HookPort=off  NonlinearTolerance=1e-4  nMaxIteration=100  ContinueOnMaxIteration=off  RestoreLinks=warning  ResistiveCurrentMeasurement=off  Frange=[0:2:500]  Ylog=off  Xlog=on  ShowGrid=off  save=off  variable=ZData  structure=0  ZoomFFT=off  StartTime=0.0  cycles=1  DisplayStyle=1  fundamental=60  FreqAxis=off  MaxFrequency=1000  frequencyindicesteady=1  RmsSteady=1  display=off
  wires:
  Current Measurement1/1 -> Scope2/3  "Blood flow of Ascending aorta"
  Voltage Measurement1/1 -> Scope11/1
  inter/1(V) -> capbianlv1/1(vl), Scope5/1
  capbianlv/1(V) -> Controlled Voltage Source/1, Scope3/1
  Voltage Measurement5/1 -> Scope7/1
  inter1/1(V) -> capbianlv/1(vl), Scope6/1
  Current Measurement2/1 -> inter1/1(vl)
  Current Measurement4/1 -> inter/1(vl)
  Voltage Measurement2/1 -> Scope10/1
  Voltage Measurement3/1 -> Scope12/1
  capbianlv1/1(V) -> Controlled Voltage Source1/1, Scope13/1
  Voltage Measurement7/1 -> Scope4/6  "Blood pressure of Ascending aorta"
  Current Measurement3/1 -> Scope9/1
  Voltage Measurement6/1 -> Scope8/1
  Voltage Measurement8/1 -> Scope4/5  "Blood pressure of Abdominal aorta Ⅰ"
  Voltage Measurement9/1 -> Scope4/3  "Blood pressure of Abdominal aorta Ⅲ"
  Voltage Measurement4/1 -> Scope4/7  "Blood pressure of Thoracic aorta"
  Voltage Measurement10/1 -> Scope4/2
  Current Measurement8/1 -> Scope2/2
  Current Measurement12/1 -> Scope1/1
  Voltage Measurement11/1 -> Scope15/2
  Voltage Measurement12/1 -> Scope15/1
  Current Measurement18/1 -> Scope16/2  "Blood flow of Inferior mesenteric artery"
  Current Measurement19/1 -> Scope16/1  "Blood flow of Superior mesenteric artery"
  Voltage Measurement13/1 -> Scope4/4  "Blood pressure of Abdominal aorta Ⅱ"
  Current Measurement32/1 -> Scope2/4  "Blood flow of Thoracic aorta"
  Current Measurement7/1 -> Scope2/5  "Blood flow of Abdominal aorta Ⅱ"
  Current Measurement31/1 -> Scope2/6  "Blood flow of Abdominal aorta Ⅲ"
  Voltage Measurement14/1 -> Scope4/1
  Current Measurement33/1 -> Scope2/1
  Current Measurement34/1 -> Scope16/3  "Blood flow of Lumbar artery"
  Current Measurement35/1 -> Scope14/8  "Blood flow of Celiac trunk"
  Current Measurement5/1 -> Scope20/1
  Current Measurement36/1 -> Scope20/3
  Current Measurement6/1 -> Scope18/8
  Current Measurement23/1 -> Scope18/7
  Current Measurement24/1 -> Scope18/6
  Current Measurement17/1 -> Scope18/5
  Current Measurement13/1 -> Scope18/4  "Blood flow of External iliac artery"
  Current Measurement14/1 -> Scope21/1
  Current Measurement15/1 -> Scope21/2
  Current Measurement40/1 -> Scope23/5
  Current Measurement47/1 -> Scope27/1
  Current Measurement38/1 -> Scope23/6
  Current Measurement48/1 -> Scope22/5
  Current Measurement58/1 -> Scope28/3
  Current Measurement52/1 -> Scope28/2
  Current Measurement59/1 -> Scope26/5
  Current Measurement49/1 -> Scope26/1
  Current Measurement46/1 -> Scope27/4
  Current Measurement26/1 -> Scope2/7
  Current Measurement62/1 -> Scope2/8
  Current Measurement39/1 -> Scope23/2
  Current Measurement37/1 -> Scope22/1
  Current Measurement51/1 -> Scope28/1
  Current Measurement60/1 -> Scope26/7
  Current Measurement61/1 -> Scope27/3
  Current Measurement63/1 -> Scope18/2  "Blood flow of Femoral artery"
  Current Measurement64/1 -> Scope2/9  "Blood flow of Abdominal aorta Ⅰ"
  Current Measurement67/1 -> Scope1/5
  Current Measurement11/1 -> Scope1/2
  Current Measurement10/1 -> Scope1/4
  Current Measurement68/1 -> Scope18/3  "Blood flow of Common iliac artery"
  Current Measurement25/1 -> Scope18/9  "Blood flow of Internal iliac artery"
  Voltage Measurement16/1 -> Scope18/10  "Blood pressure of External iliac artery"
  Current Measurement16/1 -> Scope14/1  "Blood flow of Renal artery"
  Voltage Measurement15/1 -> Scope18/11  "Blood pressure of Abdominal aorta Ⅳ"
  Voltage Measurement17/1 -> Scope18/1  "Blood pressure of Femoral artery"
  connections:
  Series RLC Branch69/RConn1 -- Series RLC Branch64/LConn1 -- Series RLC Branch65/LConn1 -- Series RLC Branch176/LConn1 -- Series RLC Branch3/LConn1
  Series RLC Branch51/RConn1 -- Series RLC Branch61/LConn1 -- Series RLC Branch49/LConn1
  Current Measurement7/RConn1 -- Current Measurement19/LConn1 -- Series RLC Branch118/LConn1
  Series RLC Branch79/LConn1 -- Series RLC Branch43/LConn1 -- Series RLC Branch81/RConn1
  Series RLC Branch72/LConn1 -- Voltage Measurement11/LConn1 -- Series RLC Branch73/RConn1 -- Series RLC Branch180/RConn1 -- Current Measurement48/RConn1 -- Current Measurement37/RConn1 -- Current Measurement38/RConn1 -- Series RLC Branch151/RConn1 -- Series RLC Branch150/RConn1
  Ground10/LConn1 -- Series RLC Branch34/RConn1
  Voltage Measurement4/LConn1 -- Series RLC Branch33/RConn1 -- Series RLC Branch34/LConn1 -- Current Measurement8/LConn1 -- Current Measurement33/LConn1
  Series RLC Branch71/LConn1 -- Series RLC Branch72/RConn1 -- Series RLC Branch70/LConn1
  Series RLC Branch128/LConn1 -- Series RLC Branch126/RConn1 -- Series RLC Branch127/LConn1
  Series RLC Branch159/LConn1 -- Series RLC Branch158/RConn1
  Series RLC Branch26/RConn1 -- Current Measurement32/LConn1 -- Series RLC Branch27/LConn1
  Series RLC Branch121/RConn1 -- Series RLC Branch122/LConn1 -- Series RLC Branch123/LConn1
  Series RLC Branch51/LConn1 -- Series RLC Branch50/RConn1
  Series RLC Branch126/LConn1 -- Series RLC Branch125/RConn1
  Series RLC Branch127/RConn1 -- Ground40/LConn1
  Series RLC Branch81/LConn1 -- Series RLC Branch80/RConn1
  Ground30/LConn1 -- Series RLC Branch92/RConn1
  Ground16/LConn1 -- Series RLC Branch27/RConn1
  Series RLC Branch119/LConn1 -- Series RLC Branch118/RConn1
  Series RLC Branch65/RConn1 -- Ground22/LConn1
  Series RLC Branch46/LConn1 -- Series RLC Branch44/RConn1
  Ground18/LConn1 -- Series RLC Branch47/RConn1
  Ground26/LConn1 -- Series RLC Branch79/RConn1
  Series RLC Branch26/LConn1 -- Series RLC Branch22/RConn1
  Series RLC Branch71/RConn1 -- Ground24/LConn1
  Series RLC Branch67/RConn1 -- Ground23/LConn1
  Series RLC Branch49/RConn1 -- Ground47/LConn1
  Series RLC Branch121/LConn1 -- Series RLC Branch120/RConn1
  Series RLC Branch31/RConn1 -- Ground9/LConn1
  Series RLC Branch32/LConn1 -- Voltage Measurement7/LConn1 -- Current Measurement1/RConn1
  Series RLC Branch124/RConn1 -- Ground39/LConn1
  Series RLC Branch122/RConn1 -- Ground38/LConn1
  Series RLC Branch133/LConn1 -- Series RLC Branch132/RConn1
  Series RLC Branch88/LConn1 -- Series RLC Branch87/RConn1
  Ground43/LConn1 -- Series RLC Branch138/RConn1
  Voltage Measurement2/LConn1 -- Series RLC Branch45/RConn1 -- Diode7/LConn1
  Diode3/LConn1 -- Series RLC Branch24/RConn1 -- Voltage Measurement1/LConn1
  Diode1/LConn1 -- Voltage Measurement5/LConn1 -- Series RLC Branch25/LConn1
  Series RLC Branch28/LConn1 -- Series RLC Branch2/LConn1 -- Series RLC Branch25/RConn1
  Series RLC Branch24/LConn1 -- Current Measurement2/LConn1 -- Diode1/RConn1
  Controlled Voltage Source1/LConn1 -- Ground14/LConn1
  Current Measurement3/LConn1 -- Diode7/RConn1 -- Series RLC Branch48/LConn1
  Current Measurement4/LConn1 -- Series RLC Branch45/LConn1 -- Diode5/RConn1
  Diode5/LConn1 -- Series RLC Branch42/RConn1
  Voltage Measurement5/LConn2 -- Ground6/LConn1
  Ground4/LConn1 -- Voltage Measurement3/LConn2
  Voltage Measurement1/LConn2 -- Ground1/LConn1
  Controlled Voltage Source1/RConn1 -- Current Measurement4/RConn1
  Ground13/LConn1 -- Series RLC Branch28/RConn1
  Current Measurement2/RConn1 -- Controlled Voltage Source/RConn1
  Ground8/LConn1 -- Controlled Voltage Source/LConn1
  Series RLC Branch9/RConn1 -- Ground49/LConn1
  Voltage Measurement4/LConn2 -- Ground2/LConn1
  Voltage Measurement7/LConn2 -- Ground3/LConn1
  Voltage Measurement2/LConn2 -- Ground7/LConn1
  Series RLC Branch10/LConn1 -- Voltage Measurement6/LConn1 -- Current Measurement3/RConn1
  Series RLC Branch11/RConn1 -- Series RLC Branch1/RConn1 -- Series RLC Branch12/LConn1
  Ground15/LConn1 -- Series RLC Branch48/RConn1
  Voltage Measurement6/LConn2 -- Ground48/LConn1
  Series RLC Branch11/LConn1 -- Series RLC Branch10/RConn1
  Ground5/LConn1 -- Series RLC Branch12/RConn1
  Series RLC Branch2/RConn1 -- Series RLC Branch1/LConn1
  Current Measurement5/RConn1 -- Series RLC Branch66/RConn1
  Voltage Measurement8/LConn2 -- Ground50/LConn1
  Voltage Measurement9/LConn2 -- Ground51/LConn1
  Series RLC Branch8/LConn1 -- Series RLC Branch66/LConn1
  Series RLC Branch9/LConn1 -- Current Measurement15/RConn1 -- Current Measurement14/RConn1 -- Voltage Measurement3/LConn1 -- Series RLC Branch42/LConn1
  Series RLC Branch91/LConn1 -- Series RLC Branch17/RConn1 -- Series RLC Branch15/LConn1
  Ground27/LConn1 -- Series RLC Branch15/RConn1
  Series RLC Branch17/LConn1 -- Series RLC Branch16/RConn1
  Series RLC Branch20/RConn1 -- Current Measurement11/LConn1 -- Series RLC Branch21/LConn1
  Series RLC Branch20/LConn1 -- Series RLC Branch19/RConn1
  Ground28/LConn1 -- Series RLC Branch21/RConn1
  Ground11/LConn1 -- Series RLC Branch7/RConn1
  Series RLC Branch6/LConn1 -- Series RLC Branch5/RConn1
  Voltage Measurement10/LConn2 -- Ground12/LConn1
  Current Measurement5/LConn1 -- Current Measurement36/LConn1 -- Current Measurement1/LConn1 -- Diode3/RConn1 -- Series RLC Branch31/LConn1
  Current Measurement8/RConn1 -- Series RLC Branch22/LConn1
  Current Measurement12/RConn1 -- Series RLC Branch16/LConn1
  Ground17/LConn1 -- Voltage Measurement11/LConn2
  Ground29/LConn1 -- Voltage Measurement12/LConn2
  Current Measurement16/LConn1 -- Voltage Measurement13/LConn1 -- Current Measurement7/LConn1 -- Current Measurement64/RConn1 -- Series RLC Branch115/LConn1
  Current Measurement17/RConn1 -- Series RLC Branch132/LConn1
  Current Measurement18/RConn1 -- Series RLC Branch125/LConn1
  Current Measurement19/RConn1 -- Series RLC Branch120/LConn1
  Series RLC Branch3/RConn1 -- Series RLC Branch8/RConn1 -- Series RLC Branch67/LConn1
  Series RLC Branch68/LConn1 -- Series RLC Branch43/RConn1
  Series RLC Branch151/LConn1 -- Series RLC Branch150/LConn1 -- Series RLC Branch68/RConn1
  Ground34/LConn1 -- Series RLC Branch74/RConn1
  Ground42/LConn1 -- Series RLC Branch94/RConn1
  Series RLC Branch93/LConn1 -- Series RLC Branch91/RConn1
  Series RLC Branch137/RConn1 -- Series RLC Branch160/LConn1 -- Series RLC Branch139/LConn1
  Series RLC Branch137/LConn1 -- Series RLC Branch136/RConn1
  Ground54/LConn1 -- Series RLC Branch139/RConn1
  Series RLC Branch142/RConn1 -- Series RLC Branch164/LConn1 -- Series RLC Branch143/LConn1
  Series RLC Branch142/LConn1 -- Series RLC Branch141/RConn1
  Ground55/LConn1 -- Series RLC Branch143/RConn1
  Current Measurement24/RConn1 -- Series RLC Branch136/LConn1
  Current Measurement25/RConn1 -- Series RLC Branch141/LConn1
  Current Measurement26/RConn1 -- Voltage Measurement14/LConn1 -- Series RLC Branch5/LConn1
  Series RLC Branch154/LConn1 -- Series RLC Branch58/LConn1 -- Series RLC Branch155/LConn1 -- Series RLC Branch153/RConn1
  Series RLC Branch153/LConn1 -- Series RLC Branch152/RConn1
  Series RLC Branch154/RConn1 -- Ground58/LConn1
  Voltage Measurement13/LConn2 -- Ground59/LConn1
  Series RLC Branch162/LConn1 -- Series RLC Branch59/LConn1 -- Series RLC Branch129/LConn1 -- Series RLC Branch159/RConn1
  Series RLC Branch165/RConn1 -- Series RLC Branch186/LConn1 -- Series RLC Branch140/LConn1 -- Series RLC Branch166/LConn1
  Series RLC Branch161/RConn1 -- Series RLC Branch60/LConn1 -- Series RLC Branch135/LConn1 -- Series RLC Branch163/LConn1
  Series RLC Branch4/LConn1 -- Series RLC Branch187/LConn1 -- Series RLC Branch168/RConn1 -- Series RLC Branch169/LConn1
  Series RLC Branch161/LConn1 -- Series RLC Branch160/RConn1
  Ground63/LConn1 -- Series RLC Branch166/RConn1
  Ground60/LConn1 -- Series RLC Branch169/RConn1
  Series RLC Branch168/LConn1 -- Series RLC Branch167/RConn1
  Ground61/LConn1 -- Series RLC Branch162/RConn1
  Ground62/LConn1 -- Series RLC Branch163/RConn1
  Series RLC Branch165/LConn1 -- Series RLC Branch164/RConn1
  Series RLC Branch138/LConn1 -- Voltage Measurement16/LConn1 -- Current Measurement13/LConn1 -- Series RLC Branch133/RConn1
  Current Measurement24/LConn1 -- Series RLC Branch172/LConn1 -- Series RLC Branch171/RConn1 -- Current Measurement17/LConn1
  Series RLC Branch124/LConn1 -- Current Measurement31/LConn1 -- Series RLC Branch119/RConn1
  Series RLC Branch33/LConn1 -- Series RLC Branch32/RConn1
  Current Measurement25/LConn1 -- Series RLC Branch174/RConn1 -- Series RLC Branch175/LConn1 -- Current Measurement26/LConn1
  Ground64/LConn1 -- Series RLC Branch172/RConn1
  Current Measurement6/RConn1 -- Current Measurement23/LConn1 -- Current Measurement68/LConn1
  Series RLC Branch170/RConn1 -- Series RLC Branch171/LConn1
  Ground65/LConn1 -- Series RLC Branch175/RConn1
  Series RLC Branch173/RConn1 -- Series RLC Branch174/LConn1
  Ground66/LConn1 -- Voltage Measurement14/LConn2
  Current Measurement23/RConn1 -- Series RLC Branch170/LConn1
  Current Measurement33/RConn1 -- Current Measurement9/LConn1
  Current Measurement6/LConn1 -- Voltage Measurement15/LConn1 -- Current Measurement34/LConn1 -- Voltage Measurement9/LConn1 -- Current Measurement31/RConn1 -- Current Measurement18/LConn1
  Current Measurement34/RConn1 -- Series RLC Branch152/LConn1
  Current Measurement35/RConn1 -- Series RLC Branch50/LConn1
  Series RLC Branch178/LConn1 -- Series RLC Branch176/RConn1 -- Series RLC Branch179/RConn1
  Series RLC Branch178/RConn1 -- Ground67/LConn1
  Series RLC Branch179/LConn1 -- Series RLC Branch177/LConn1
  Current Measurement36/RConn1 -- Series RLC Branch177/RConn1
  Series RLC Branch7/LConn1 -- Current Measurement62/LConn1 -- Voltage Measurement10/LConn1 -- Series RLC Branch6/RConn1
  Current Measurement14/LConn1 -- Series RLC Branch70/RConn1
  Current Measurement15/LConn1 -- Series RLC Branch69/LConn1
  Series RLC Branch44/LConn1 -- Current Measurement32/RConn1 -- Current Measurement35/LConn1 -- Voltage Measurement8/LConn1
  Current Measurement37/LConn1 -- Series RLC Branch18/RConn1
  Current Measurement39/LConn1 -- Series RLC Branch14/RConn1
  Series RLC Branch94/LConn1 -- Series RLC Branch55/LConn1 -- Series RLC Branch14/LConn1 -- Series RLC Branch93/RConn1
  Current Measurement40/LConn1 -- Series RLC Branch55/RConn1
  Current Measurement47/LConn1 -- Current Measurement46/RConn1 -- Current Measurement61/RConn1
  Current Measurement49/LConn1 -- Current Measurement59/RConn1 -- Current Measurement60/RConn1
  Current Measurement51/LConn1 -- Series RLC Branch155/RConn1
  Current Measurement39/RConn1 -- Current Measurement38/LConn1 -- Current Measurement40/RConn1
  Current Measurement48/LConn1 -- Series RLC Branch54/RConn1
  Current Measurement58/LConn1 -- Current Measurement52/RConn1 -- Current Measurement51/RConn1
  Current Measurement52/LConn1 -- Series RLC Branch58/RConn1
  Current Measurement59/LConn1 -- Series RLC Branch129/RConn1
  Current Measurement60/LConn1 -- Series RLC Branch59/RConn1
  Current Measurement46/LConn1 -- Series RLC Branch60/RConn1
  Current Measurement61/LConn1 -- Series RLC Branch135/RConn1
  Current Measurement63/LConn1 -- Voltage Measurement17/LConn1 -- Current Measurement13/RConn1
  Series RLC Branch88/RConn1 -- Series RLC Branch73/LConn1 -- Series RLC Branch180/LConn1 -- Series RLC Branch92/LConn1
  Current Measurement63/RConn1 -- Series RLC Branch158/LConn1
  Series RLC Branch46/RConn1 -- Current Measurement64/LConn1 -- Series RLC Branch47/LConn1
  Current Measurement12/LConn1 -- Current Measurement67/LConn1 -- Current Measurement9/RConn1 -- Current Measurement10/LConn1
  Series RLC Branch80/LConn1 -- Current Measurement10/RConn1
  Series RLC Branch85/LConn1 -- Series RLC Branch84/RConn1
  Ground25/LConn1 -- Series RLC Branch78/RConn1
  Current Measurement67/RConn1 -- Series RLC Branch84/LConn1
  Series RLC Branch54/LConn1 -- Current Measurement11/RConn1 -- Series RLC Branch18/LConn1
  Current Measurement68/RConn1 -- Series RLC Branch173/LConn1
  Series RLC Branch167/LConn1 -- Current Measurement62/RConn1
  Series RLC Branch78/LConn1 -- Series RLC Branch19/LConn1 -- Series RLC Branch87/LConn1 -- Series RLC Branch85/RConn1
  Voltage Measurement16/LConn2 -- Ground20/LConn1
  Series RLC Branch117/LConn1 -- Series RLC Branch114/LConn1 -- Series RLC Branch116/RConn1
  Series RLC Branch112/RConn1 -- Series RLC Branch113/LConn1 -- Series RLC Branch110/LConn1
  Series RLC Branch116/LConn1 -- Series RLC Branch115/RConn1
  Ground36/LConn1 -- Series RLC Branch113/RConn1
  Series RLC Branch112/LConn1 -- Series RLC Branch111/RConn1
  Series RLC Branch111/LConn1 -- Current Measurement16/RConn1
  Ground37/LConn1 -- Series RLC Branch117/RConn1
  Series RLC Branch61/RConn1 -- Current Measurement47/RConn1 -- Current Measurement49/RConn1 -- Series RLC Branch186/RConn1 -- Series RLC Branch140/RConn1 -- Series RLC Branch187/RConn1 -- Series RLC Branch4/RConn1 -- Current Measurement58/RConn1 -- Series RLC Branch128/RConn1 -- Series RLC Branch123/RConn1 -- Series RLC Branch114/RConn1 -- Series RLC Branch110/RConn1 -- Voltage Measurement12/LConn1 -- Series RLC Branch64/RConn1
  Voltage Measurement15/LConn2 -- Ground19/LConn1
  Voltage Measurement17/LConn2 -- Ground21/LConn1

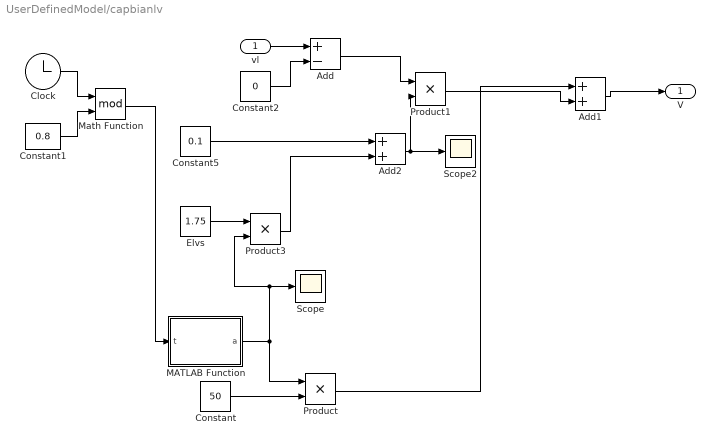
== system UserDefinedModel/capbianlv ==
  vl : Inport
  Add : Sum  Inputs=+-
  Add1 : Sum
  Add2 : Sum
  Clock : Clock
  Constant : Constant  Value=50
  Constant1 : Constant  Value=0.8
  Constant2 : Constant  Value=0
  Constant5 : Constant  Value=0.1
  Elvs : Constant  Value=1.75
  MATLAB Function : MATLAB Function  TreatAsAtomicUnit=on
  Math Function : Math  Operator=mod  SignedPower=on
  Product : Product
  Product1 : Product
  Product3 : Product
  Scope : Scope
  Scope2 : Scope
  V : Outport  VectorParamsAs1DForOutWhenUnconnected=off
  wires:
  Constant1/1 -> Math Function/2
  Math Function/1 -> MATLAB Function/1(t)
  Clock/1 -> Math Function/1
  MATLAB Function/1(a) -> Product3/2, Scope/1, Product/1
  Constant/1 -> Product/2
  Constant2/1 -> Add/2
  Add1/1 -> V/1
  Elvs/1 -> Product3/1
  Constant5/1 -> Add2/1
  Product/1 -> Add1/1
  vl/1 -> Add/1
  Add/1 -> Product1/1
  Add2/1 -> Scope2/1, Product1/2
  Product1/1 -> Add1/2
  Product3/1 -> Add2/2
